simulink model "MIMO_StabilizedSystem"  (R2025b)
settings: Solver=VariableStepAuto  StartTime=0.0  StopTime=10.0  RelTol=1e-3
undefined symbols (not defined in the file or in its folder): linmodel
libraries: eeLuenbergerObserver x1, Drone_MIMO_Simple_Model x1
settings Model: Creator=Alek  LastModifiedBy=Alek

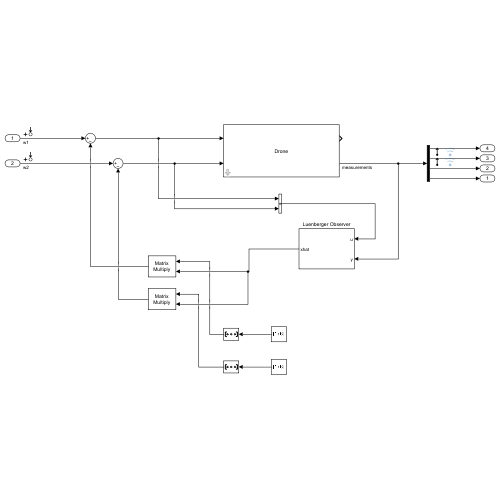
[thumbnail: Simulink's stored preview of the top-level diagram]
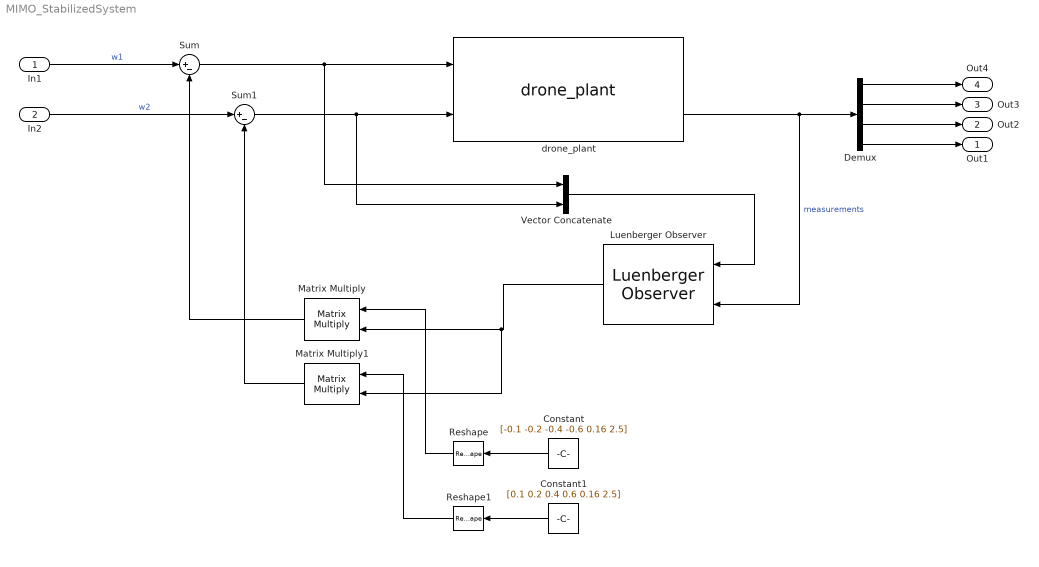
== system MIMO_StabilizedSystem ==
  In1 : Inport
  In2 : Inport  Port=2
  Constant : Constant  Value=[-0.1 -0.2 -0.4 -0.6 0.16 2.5]
  Constant1 : Constant  Value=[0.1 0.2 0.4 0.6 0.16 2.5]
  Demux : Demux
  Luenberger Observer : eeLuenbergerObserver/Luenberger Observer  StateSpaceType=Continuous-time  Ad=linmodel.A  Bd=linmodel.B  Cd=linmodel.C  Dd=linmodel.D  A=linmodel.A  B=linmodel.B  C=linmodel.C  D=linmodel.D  ObserverDesign=Desired eigenvalues  Ld=1  DesiredEigenvalues=[-2 -3 -4 -6 -7 -8]  x0=[0; 0; 0; 0; 0; 0]  Tsd=0.001  Ts=-1
      settings: LibrarySourceBlock=ee_sl_lib/Observers/Luenberger Observer
  Matrix Multiply : Product  Multiplication=Matrix(*)
  Matrix Multiply1 : Product  Multiplication=Matrix(*)
  Reshape : Reshape  OutputDimensionality=Row vector (2-D)
  Reshape1 : Reshape  OutputDimensionality=Row vector (2-D)
  Sum : Sum  Inputs=|+-
  Sum1 : Sum  Inputs=|+-
  Vector Concatenate : Concatenate
  drone_plant : Drone_MIMO_Simple_Model/drone_plant  kf=1e-5  m=0.5  l=1e-2  Irod=6.6666e-5
      settings: SourceProductName=DroneLibrary
  Out1 : Outport
  Out2 : Outport  Port=2
  Out3 : Outport  Port=3
  Out4 : Outport  Port=4
  wires:
  drone_plant/2 -> Luenberger Observer/2, Demux/1  "measurements"
  Vector Concatenate/1 -> Luenberger Observer/1
  Constant/1 -> Reshape/1
  Reshape/1 -> Matrix Multiply/1
  In1/1 -> Sum/1  "w1"
  Sum/1 -> Vector Concatenate/1, drone_plant/1
  Matrix Multiply/1 -> Sum/2
  In2/1 -> Sum1/1  "w2"
  Sum1/1 -> Vector Concatenate/2, drone_plant/2
  Constant1/1 -> Reshape1/1
  Reshape1/1 -> Matrix Multiply1/1
  Luenberger Observer/1 -> Matrix Multiply1/2, Matrix Multiply/2
  Matrix Multiply1/1 -> Sum1/2
  Demux/2 -> Out3/1
  Demux/1 -> Out4/1
  Demux/4 -> Out1/1
  Demux/3 -> Out2/1
